simulink model "simSTA"  (R2023b)
settings: Solver=ode45  StartTime=0.0  StopTime=100.0  RelTol=1e-3
values from neighbouring files (symbols this model uses):
  alphadot_not0 = omega_1*sqrt(gamma_1/2)    [runSTA.m]
  D_d = eye(6)*3    [runSTA.m]
  dragcoeff = [C_d_1, C_d_4, C_d_C, C_d_L, beta, gamma]    [runSTA.m]
  epsilon = 1    [runSTA.m]
  G_d = eye(6)*0.5    [runSTA.m]
  lambda_SM = 15    [runSTA.m]
  M_d = eye(6)*4    [runSTA.m]
  pos_init = [0 (2*0.77*cos(pi/4)+1) 0]    [runSTA.m]
  quat_init = eul2quat([0 0 pi],'XYZ')    [runSTA.m]
  theta_init = [0 pi/4 0 pi/4 pi/4 0 pi/4 0]    [runSTA.m]
  x_init = [pos_init quat_init theta_init zeta_init]'    [runSTA.m]
undefined symbols (not defined in the file or in its folder): pp, snake
libraries: dspindex x2, cstblocks x1
settings Model: Creator=sarava  LastModifiedBy=asker
settings SolverCC: MaxConsecutiveMinStep=3  AlgebraicLoopSolver=TrustRegion
settings DataIOCC: ReturnWorkspaceOutputs=off
settings DebuggingCC: UnconnectedInputMsg=warning  UnconnectedOutputMsg=warning  UnconnectedLineMsg=warning  ArithmeticOperatorsInVariantConditions=warning
settings ModelReferenceCC: EnableRefExpFcnMdlSchedulingChecks=on
settings SFSimCC: SimUseLocalCustomCode=off  CustomCodeUndefinedFunction=UseInterfaceOnly
settings RTWCC: RTWUseLocalCustomCode=off  BuildConfiguration=Faster Runs

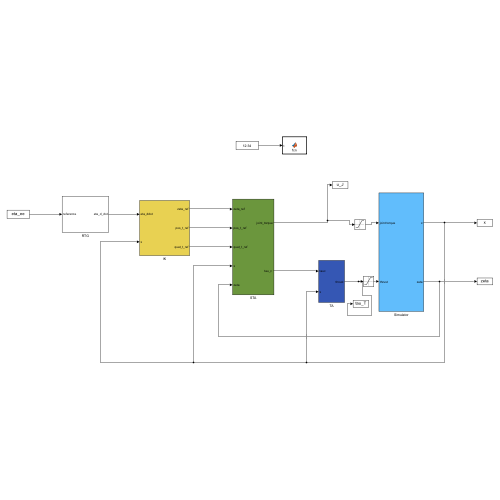
[thumbnail: Simulink's stored preview of the top-level diagram]
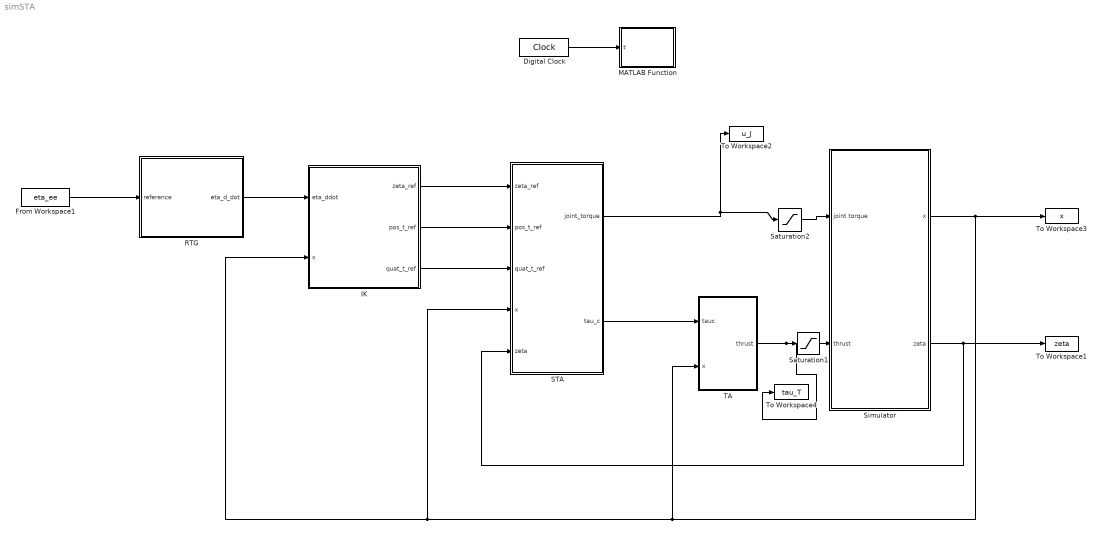
== system simSTA ==
  Digital Clock : DigitalClock
  From Workspace1 : FromWorkspace  VariableName=eta_ee
  IK : Subsystem
  MATLAB Function : MATLAB Function  TreatAsAtomicUnit=on
  RTG : Subsystem
  STA : Subsystem
  Saturation1 : Saturate  UpperLimit=20  LowerLimit=-20  ZeroCross=off
  Saturation2 : Saturate  UpperLimit=10  LowerLimit=-10  ZeroCross=off
  Simulator : Subsystem
  TA : Subsystem
  To Workspace1 : ToWorkspace  VariableName=zeta  SaveFormat=Timeseries  SampleTime=-1
  To Workspace2 : ToWorkspace  VariableName=u_J  SaveFormat=Timeseries  SampleTime=-1
  To Workspace3 : ToWorkspace  VariableName=x  SaveFormat=Timeseries  SampleTime=-1
  To Workspace4 : ToWorkspace  VariableName=tau_T  SaveFormat=Timeseries  SampleTime=-1
  wires:
  RTG/1(eta_d_dot) -> IK/1(eta_ddot)
  TA/1(thrust) -> To Workspace4/1, Saturation1/1
  Digital Clock/1 -> MATLAB Function/1(t)
  STA/1(joint_torque) -> Saturation2/1, To Workspace2/1
  From Workspace1/1 -> RTG/1(reference)
  STA/2("tau_c ") -> TA/1("tauc ")
  IK/1(zeta_ref) -> STA/1(zeta_ref)
  Simulator/2(zeta) -> STA/5("zeta "), To Workspace1/1
  IK/2(pos_t_ref) -> STA/2(pos_t_ref)
  Simulator/1(x) -> STA/4("x "), IK/2(x), TA/2("x "), To Workspace3/1
  IK/3(quat_t_ref) -> STA/3(quat_t_ref)
  Saturation2/1 -> Simulator/1(joint torque)
  Saturation1/1 -> Simulator/2(thrust)

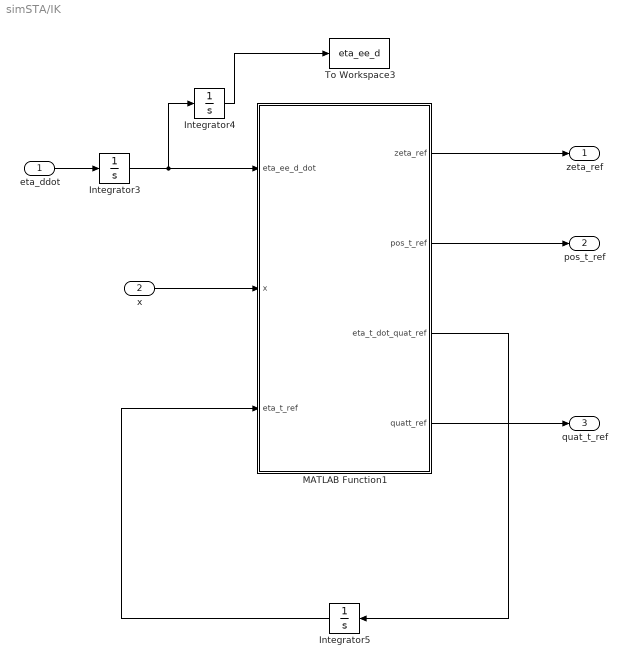
== system simSTA/IK ==
  eta_ddot : Inport
  x : Inport  Port=2
  Integrator3 : Integrator
  Integrator4 : Integrator
  Integrator5 : Integrator  InitialCondition=[pos_init quat_init]'
  MATLAB Function1 : MATLAB Function  TreatAsAtomicUnit=on
  To Workspace3 : ToWorkspace  VariableName=eta_ee_d  SaveFormat=Timeseries  SampleTime=-1
  zeta_ref : Outport  VectorParamsAs1DForOutWhenUnconnected=off
  pos_t_ref : Outport  Port=2  VectorParamsAs1DForOutWhenUnconnected=off
  quat_t_ref : Outport  Port=3  VectorParamsAs1DForOutWhenUnconnected=off
  wires:
  MATLAB Function1/1(zeta_ref) -> zeta_ref/1
  x/1 -> MATLAB Function1/2(x)
  MATLAB Function1/2(pos_t_ref) -> pos_t_ref/1
  MATLAB Function1/3(eta_t_dot_quat_ref) -> Integrator5/1
  Integrator4/1 -> To Workspace3/1
  Integrator5/1 -> MATLAB Function1/3(eta_t_ref)
  MATLAB Function1/4(quatt_ref) -> quat_t_ref/1
  eta_ddot/1 -> Integrator3/1
  Integrator3/1 -> Integrator4/1, MATLAB Function1/1(eta_ee_d_dot)

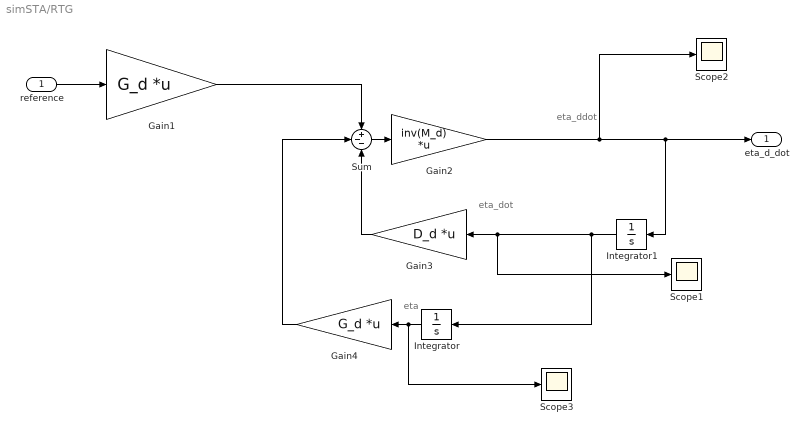
== system simSTA/RTG ==
  note: eta_dot
  note: eta
  note: eta_ddot
  reference : Inport
  Gain1 : Gain  Gain=G_d  Multiplication=Matrix(K*u) (u vector)
  Gain2 : Gain  Gain=inv(M_d)  Multiplication=Matrix(K*u) (u vector)
  Gain3 : Gain  Gain=D_d  Multiplication=Matrix(K*u) (u vector)
  Gain4 : Gain  Gain=G_d  Multiplication=Matrix(K*u) (u vector)
  Integrator : Integrator
  Integrator1 : Integrator
  Scope1 : Scope
  Scope2 : Scope
  Scope3 : Scope
  Sum : Sum  Inputs=+--
  eta_d_dot : Outport  VectorParamsAs1DForOutWhenUnconnected=off
  wires:
  Gain2/1 -> Scope2/1, eta_d_dot/1, Integrator1/1
  Gain1/1 -> Sum/1
  Sum/1 -> Gain2/1
  reference/1 -> Gain1/1
  Integrator1/1 -> Integrator/1, Scope1/1, Gain3/1
  Integrator/1 -> Scope3/1, Gain4/1
  Gain3/1 -> Sum/3
  Gain4/1 -> Sum/2

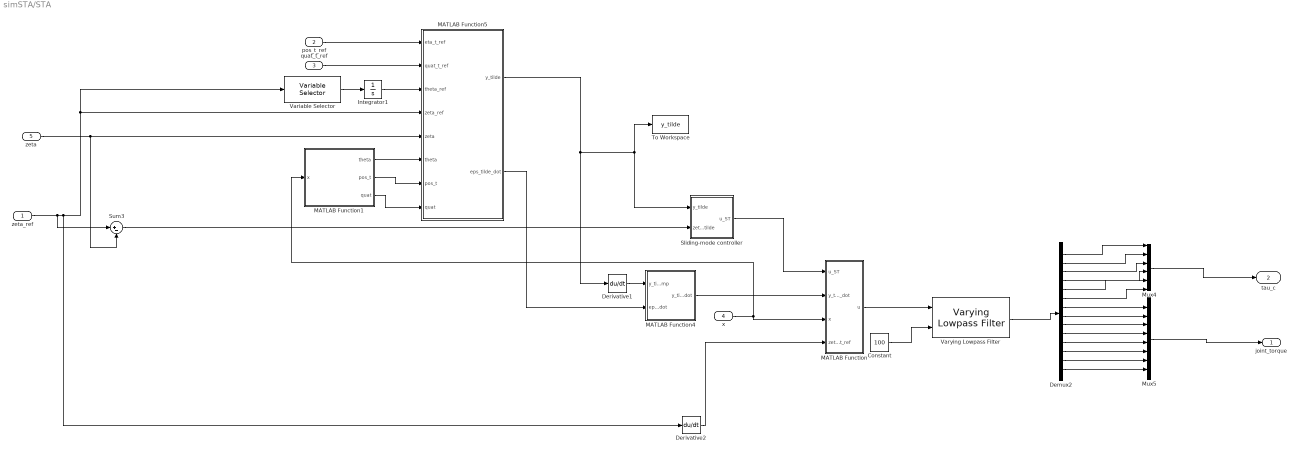
== system simSTA/STA ==
  zeta_ref : Inport
  pos_t_ref : Inport  Port=2
  quat_t_ref : Inport  Port=3
  "x " : Inport  Port=4
  "zeta " : Inport  Port=5
  Constant : Constant  Value=100
  Demux2 : Demux  Outputs=14
  Derivative1 : Derivative  CoefficientInTFapproximation=10
  Derivative2 : Derivative  CoefficientInTFapproximation=10
  Integrator1 : Integrator  InitialCondition=theta_init
  MATLAB Function : MATLAB Function  TreatAsAtomicUnit=on
  MATLAB Function1 : MATLAB Function  TreatAsAtomicUnit=on
  MATLAB Function4 : MATLAB Function  TreatAsAtomicUnit=on
  MATLAB Function5 : MATLAB Function  TreatAsAtomicUnit=on
  Mux4 : Mux  Inputs=6
  Mux5 : Mux  Inputs=8
  "Sliding-mode controller " : Subsystem
  Sum3 : Sum  Inputs=|+-
  To Workspace : ToWorkspace  VariableName=y_tilde  SaveFormat=Timeseries  SampleTime=-1
  Variable Selector : dspindex/Variable Selector  NumInputs=1  rowsOrCols=Rows  IdxMode=Fixed  Elements=7:14  ZerOneIdxMode=One-based  errmode=Clip Index  FillMode=on  FillValues=0
  Varying Lowpass Filter : cstblocks/Linear Parameter Varying/Varying Lowpass Filter  N=2
  joint_torque : Outport  VectorParamsAs1DForOutWhenUnconnected=off
  "tau_c " : Outport  Port=2  VectorParamsAs1DForOutWhenUnconnected=off
  wires:
  Demux2/13 -> Mux5/7
  Demux2/14 -> Mux5/8
  Demux2/8 -> Mux5/2
  Demux2/11 -> Mux5/5
  Demux2/10 -> Mux5/4
  Demux2/4 -> Mux4/4
  Demux2/2 -> Mux4/2
  Demux2/1 -> Mux4/1
  Demux2/12 -> Mux5/6
  Demux2/3 -> Mux4/3
  Demux2/7 -> Mux5/1
  Demux2/6 -> Mux4/6
  Demux2/5 -> Mux4/5
  Demux2/9 -> Mux5/3
  zeta_ref/1 -> Variable Selector/1, MATLAB Function5/4(zeta_ref), Derivative2/1, Sum3/1
  Mux5/1 -> joint_torque/1
  Mux4/1 -> "tau_c "/1
  Sum3/1 -> "Sliding-mode controller "/2(zeta_tilde)
  "x "/1 -> MATLAB Function/3(x), MATLAB Function1/1(x)
  "Sliding-mode controller "/1(u_ST) -> MATLAB Function/1(u_ST)
  Derivative1/1 -> MATLAB Function4/1(y_tilde_dot_temp)
  MATLAB Function5/1(y_tilde) -> Derivative1/1, To Workspace/1, "Sliding-mode controller "/1(y_tilde)
  MATLAB Function5/2(eps_tilde_dot) -> MATLAB Function4/2(eps_tilde_dot)
  MATLAB Function4/1(y_tilde_dot) -> MATLAB Function/2(y_tilde_dot)
  Derivative2/1 -> MATLAB Function/4(zeta_dot_ref)
  Variable Selector/1 -> Integrator1/1
  Integrator1/1 -> MATLAB Function5/3(theta_ref)
  pos_t_ref/1 -> MATLAB Function5/1(eta_t_ref)
  quat_t_ref/1 -> MATLAB Function5/2(quat_t_ref)
  MATLAB Function/1(u) -> Varying Lowpass Filter/1
  "zeta "/1 -> MATLAB Function5/5(zeta), Sum3/2
  MATLAB Function1/3(quat) -> MATLAB Function5/8(quat)
  MATLAB Function1/2(pos_t) -> MATLAB Function5/7(pos_t)
  MATLAB Function1/1(theta) -> MATLAB Function5/6(theta)
  Varying Lowpass Filter/1 -> Demux2/1
  Constant/1 -> Varying Lowpass Filter/2

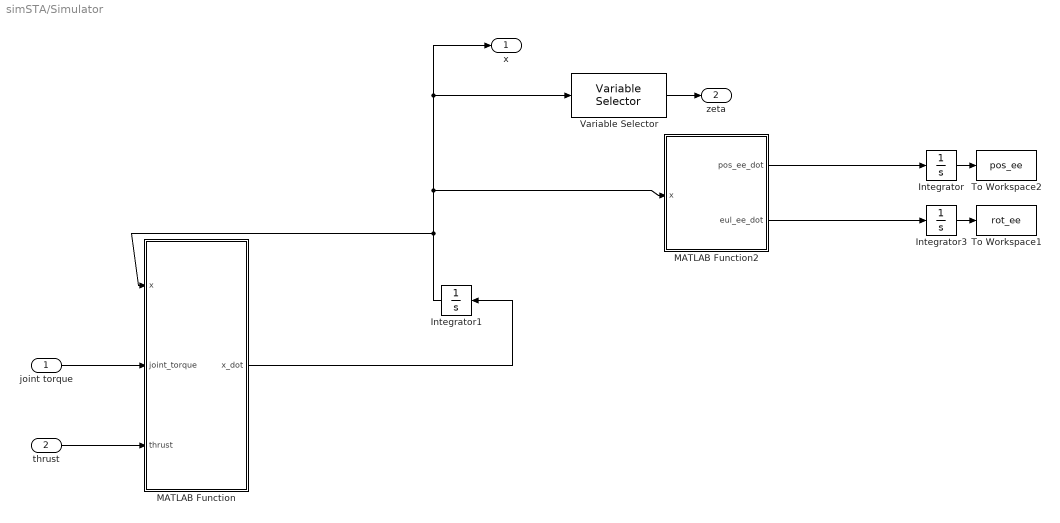
== system simSTA/Simulator ==
  joint torque : Inport
  thrust : Inport  Port=2
  Integrator : Integrator
  Integrator1 : Integrator  InitialCondition=x_init
  Integrator3 : Integrator
  MATLAB Function : MATLAB Function  TreatAsAtomicUnit=on
  MATLAB Function2 : MATLAB Function  TreatAsAtomicUnit=on
  To Workspace1 : ToWorkspace  VariableName=rot_ee  SaveFormat=Timeseries  SampleTime=-1
  To Workspace2 : ToWorkspace  VariableName=pos_ee  SaveFormat=Timeseries  SampleTime=-1
  Variable Selector : dspindex/Variable Selector  NumInputs=1  rowsOrCols=Rows  IdxMode=Fixed  Elements=16:29  ZerOneIdxMode=One-based  errmode=Clip Index  FillMode=on  FillValues=0
  x : Outport  VectorParamsAs1DForOutWhenUnconnected=off
  zeta : Outport  Port=2  VectorParamsAs1DForOutWhenUnconnected=off
  wires:
  joint torque/1 -> MATLAB Function/2(joint_torque)
  thrust/1 -> MATLAB Function/3(thrust)
  Variable Selector/1 -> zeta/1
  MATLAB Function/1(x_dot) -> Integrator1/1
  Integrator1/1 -> Variable Selector/1, x/1, MATLAB Function2/1(x), MATLAB Function/1(x)
  Integrator/1 -> To Workspace2/1
  MATLAB Function2/1(pos_ee_dot) -> Integrator/1
  MATLAB Function2/2(eul_ee_dot) -> Integrator3/1
  Integrator3/1 -> To Workspace1/1

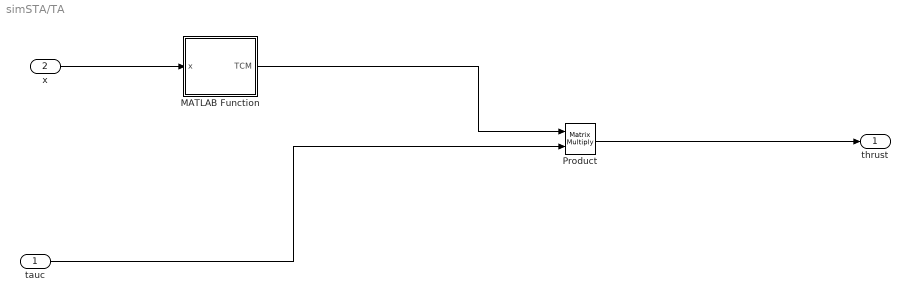
== system simSTA/TA ==
  "tauc " : Inport
  "x " : Inport  Port=2
  MATLAB Function : MATLAB Function  TreatAsAtomicUnit=on
  Product : Product  Multiplication=Matrix(*)
  thrust : Outport  VectorParamsAs1DForOutWhenUnconnected=off
  wires:
  "x "/1 -> MATLAB Function/1(x)
  MATLAB Function/1(TCM) -> Product/1
  "tauc "/1 -> Product/2
  Product/1 -> thrust/1

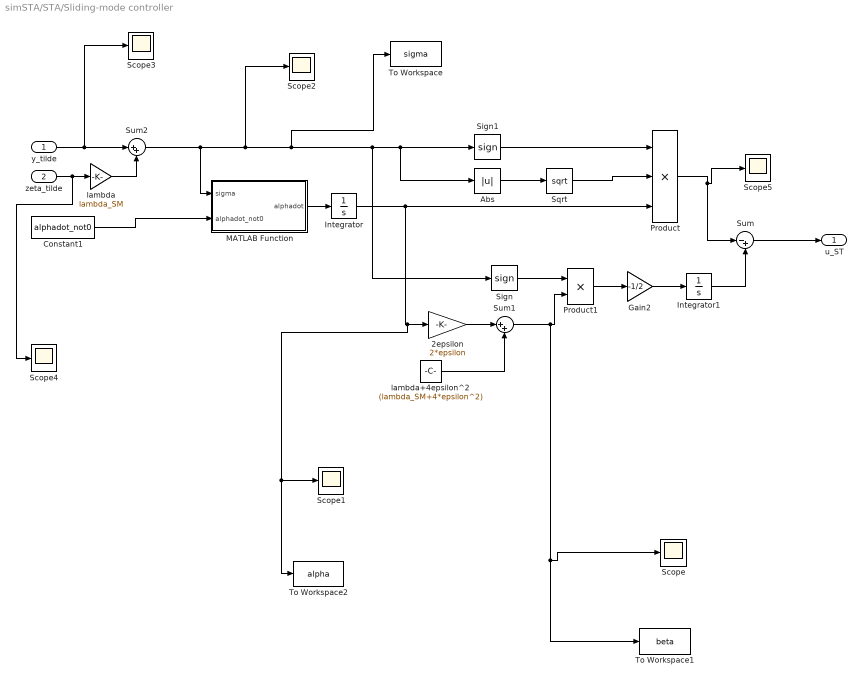
== system simSTA/STA/Sliding-mode controller  ==
  y_tilde : Inport
  zeta_tilde : Inport  Port=2
  2epsilon : Gain  Gain=2*epsilon
  Abs : Abs  ZeroCross=off  SaturateOnIntegerOverflow=off
  Constant1 : Constant  Value=alphadot_not0  SampleTime=0.001
  Gain2 : Gain  Gain=-1/2
  Integrator : Integrator
  Integrator1 : Integrator
  MATLAB Function : MATLAB Function  TreatAsAtomicUnit=on
  Product : Product  Inputs=3
  Product1 : Product
  Scope{,1..5} (6 alike) : Scope
  Sign : Signum  ZeroCross=off
  Sign1 : Signum  ZeroCross=off
  Sqrt : Sqrt
  Sum : Sum  Inputs=|-+
  Sum1 : Sum  Inputs=|++
  Sum2 : Sum  Inputs=|++
  To Workspace : ToWorkspace  VariableName=sigma  SaveFormat=Timeseries  SampleTime=-1
  To Workspace1 : ToWorkspace  VariableName=beta  SaveFormat=Timeseries  SampleTime=-1
  To Workspace2 : ToWorkspace  VariableName=alpha  SaveFormat=Timeseries  SampleTime=-1
  lambda : Gain  Gain=lambda_SM
  lambda+4epsilon^2 : Constant  Value=(lambda_SM+4*epsilon^2)
  u_ST : Outport  VectorParamsAs1DForOutWhenUnconnected=off
  wires:
  zeta_tilde/1 -> Scope4/1, lambda/1
  Sum/1 -> u_ST/1
  Product/1 -> Scope5/1, Sum/1
  2epsilon/1 -> Sum1/1
  Sign/1 -> Product1/1
  MATLAB Function/1(alphadot) -> Integrator/1
  Constant1/1 -> MATLAB Function/2(alphadot_not0)
  lambda/1 -> Sum2/2
  y_tilde/1 -> Scope3/1, Sum2/1
  Sign1/1 -> Product/1
  Sqrt/1 -> Product/2
  Abs/1 -> Sqrt/1
  Integrator1/1 -> Sum/2
  Gain2/1 -> Integrator1/1
  Product1/1 -> Gain2/1
  Integrator/1 -> Scope1/1, To Workspace2/1, 2epsilon/1, Product/3
  lambda+4epsilon^2/1 -> Sum1/2
  Sum1/1 -> Scope/1, To Workspace1/1, Product1/2
  Sum2/1 -> Scope2/1, To Workspace/1, Sign/1, Abs/1, Sign1/1, MATLAB Function/1(sigma)

== matlab function simSTA/TA/MATLAB Function ==
  data: TCM output; x input; snake parameter
function TCM = fcn(x , snake)
quat      =  x(4:7);
theta     =  x(8 : 6+snake.n);
[~, J]    =  comp_rot_jac(quat,theta,snake);
B        =  comp_TCM(J,snake);
TCM_t=B(1:6,:);
TCM=transpose(TCM_t)/(TCM_t*transpose(TCM_t));

== matlab function simSTA/STA/Sliding-mode controller /MATLAB Function ==
  data: sigma input; alphadot output; alphadot_not0 input; alpha_m parameter
function alphadot = fcn(sigma,alphadot_not0,alpha_m)

alphadot=zeros(14,1);

for count=1:14
    if (abs(sigma(count))>alpha_m)
        alphadot(count)=alphadot_not0(count);
    else
        alphadot(count)=0;
    end
end

== matlab function simSTA/STA/MATLAB Function4 ==
  data: y_tilde_dot_temp input; eps_tilde_dot input; y_tilde_dot output
function y_tilde_dot = calc_estdot(y_tilde_dot_temp,eps_tilde_dot)

y_tilde_dot=[y_tilde_dot_temp(1:3);eps_tilde_dot;y_tilde_dot_temp(7:14)];
end

== matlab function simSTA/IK/MATLAB Function1 ==
  data: eta_ee_d_dot input; x input; eta_t_ref input; zeta_ref output; snake parameter; pos_t_ref output; eta_t_dot_quat_ref output; quatt_ref output
function [zeta_ref , pos_t_ref,eta_t_dot_quat_ref, quatt_ref] = fucn(eta_ee_d_dot,x,eta_t_ref, snake)
quat      =  x(4:7);
theta     =  x(8 : 6+snake.n);
[R, J_t]    =  comp_rot_jac(quat,theta,snake);


eul_ee=rotm2eul(R(:,:,10), 'XYZ')';

Jinv=Jinv_fromeul(eul_ee);
J=[R(:,:,10) zeros(3); zeros(3) Jinv]*J_t(:,:,10);

zeta_ref=J'/(J*J'+0.0001*eye(6))*(eta_ee_d_dot);%+K*sigma_tilde);
eta_ee_ref_dot=J*zeta_ref;



quatt_ref=eta_t_ref(4:7);
pos_t_ref=eta_t_ref(1:3);
R_tail=quat2rotm(quatt_ref');

pos_t_dot   =  R_tail(:,:,1)*zeta_ref(1:3);  
quat_t_dot  =  TransAngQ(quatt_ref)*zeta_ref(4:6)+1*(1-quatt_ref'*quatt_ref)*quatt_ref; 

eta_t_dot_quat_ref=[pos_t_dot; quat_t_dot];
end

== matlab function simSTA/STA/MATLAB Function5 ==
  data: y_tilde output; eta_t_ref input; quat_t_ref input size=4; theta_ref input; eps_tilde_dot output; zeta_ref input; zeta input; theta input; pos_t input; quat input
function [y_tilde,eps_tilde_dot] = dyn(eta_t_ref, quat_t_ref, theta_ref, zeta_ref,zeta,theta,pos_t,quat)


theta_tilde=theta_ref-theta;
pos_t_ref=eta_t_ref(1:3);
pos_tilde=quat2rotm(quat')*(pos_t_ref-pos_t);




quat_tilde=quat(1)*quat_t_ref(2:4)-quat_t_ref(1)*quat(2:4)+cross(quat_t_ref(2:4),quat(2:4));
eta_tilde = quat(1) * quat_t_ref (1) + quat_t_ref(2:4)'*quat(2:4);
if eta_tilde < 0
quat_tilde = - quat_tilde ;
end


y_tilde=[pos_tilde;quat_tilde; theta_tilde];

nu2_tilde=zeta_ref(4:6)-zeta(4:6);
eps_tilde_dot=0.5*eta_tilde*nu2_tilde + 0.5*skew(quat_tilde)*nu2_tilde;


end

== matlab function simSTA/STA/MATLAB Function1 ==
  data: x input; theta output; pos_t output; quat output; snake parameter
function [theta,pos_t,quat] = dyn(x,snake)
pos_t       =  x(1:3);
quat      =  x(4:7);
theta     =  x(8 : 6+snake.n);


end

== matlab function simSTA/MATLAB Function ==
  data: t input
function fcn(t)
%#codegen
coder.extrinsic('fprintf');
persistent firstTime

if isempty(firstTime)
    firstTime = false;
    fprintf('Starting Now\n');
end

fprintf('time = %.4f\n',t);

== matlab function simSTA/Simulator/MATLAB Function ==
  data: x input; x_dot output; joint_torque input size=8; thrust input size=10; pp parameter; snake parameter; dragcoeff parameter
function x_dot  = dyn(x,joint_torque,thrust , pp, snake, dragcoeff)

pos       =  x(1:3);
quat      =  x(4:7);
theta     =  x(8 : 6+snake.n);
zeta      =  x(7+snake.n : 11+2*snake.n);
%Compute rotation matrices and jacobians
[Rcdg,Jcdg]=comp_rot_jac_mcdg(quat,theta,snake);
%Compute mass matrix
M         =  comp_mass(Jcdg,snake);

%Compute relative velocity to take into account the effect of current
velc_h    =  Rcdg(:,:,1)'*pp.velc;
nu        =  zeta(1:6);
zeta(1:3) =  zeta(1:3)-velc_h;

%Compute coriolis, drag, and hydrostatic terms with the relative velocity
[c, d, g] =  comp_cdg(Jcdg,Rcdg,theta,snake,pp,dragcoeff,zeta);
%Compute the thrust-configuration matrix
B         =  comp_TCM(Jcdg,snake);


%Compute the relative acceleration
zeta_dot      =  M\([B [zeros(6,8); eye(8)]]*[thrust;joint_torque]-c-d-g);% -c-d-g

%Remove the effect of current
zeta_dot(1:3) = zeta_dot(1:3)-cross(nu(4:6),velc_h);
%Compute the time derivatives of position and orientation
pos_dot   =  Rcdg(:,:,1)*nu(1:3);  
quat_dot  =  TransAngQ(quat)*nu(4:6)+1*(1-quat'*quat)*quat; 
%Assemble derivative of the state vector
x_dot = [pos_dot ; quat_dot ; zeta(7:snake.n+5) ; zeta_dot];
end

== matlab function simSTA/STA/MATLAB Function ==
  data: u_ST input; y_tilde_dot input; x input; zeta_dot_ref input; pp parameter; snake parameter; dragcoeff parameter; u output; lambda_SM parameter
function u  = dyn(u_ST,y_tilde_dot,x, zeta_dot_ref, pp, snake, dragcoeff,lambda_SM)



pos       =  x(1:3);
quat      =  x(4:7);
theta     =  x(8 : 6+snake.n);
zeta      =  x(7+snake.n : 11+2*snake.n);
[R, J]    =  comp_rot_jac(quat,theta,snake);
M         =  comp_mass(J,snake);
[c, ~, g] =  comp_cdg(J,R,theta,snake,pp,dragcoeff,zeta);
B=comp_TCM(J,snake);
B_u=[eye(6,6) zeros(6,8); B(7:end,:)*pinv(B(1:6,:)) eye(8)];

u=pinv(B_u)*(c+g+M*inv(lambda_SM)*(lambda_SM*zeta_dot_ref-u_ST+y_tilde_dot));%pinv(B_u)*(c+g-M*(inv(lambda_SM)*(u_ST-y_tilde_dot))+zeta_dot_ref);
end

== matlab function simSTA/Simulator/MATLAB Function2 ==
  data: pos_ee_dot output; x input; snake parameter; eul_ee_dot output
function [pos_ee_dot, eul_ee_dot] = snake2points(x,snake)
   quat         = x(4:7);
   theta        = x(8 : 6+snake.n);
    zeta      =  x(7+snake.n : 11+2*snake.n);

   [R,J]=comp_rot_jac(quat,theta,snake);
  
   eul_ee=rotm2eul(R(:,:,10), 'XYZ')';
   Jinv=Jinv_fromeul(eul_ee);
   eta_ee_dot=[R(:,:,10) zeros(3); zeros(3) Jinv]*J(:,:,10)*zeta;
   x_ee_dot=[R(:,:,10) zeros(3); zeros(3) R(:,:,10)]*J(:,:,10)*zeta;
   pos_ee_dot=x_ee_dot(1:3);
   omega_ee=x_ee_dot(4:6);
   eul_ee_dot=eta_ee_dot(4:6);
end
